simulink model "RotatingMasses_Template"  (R2019b)
settings: Solver=ode1  StartTime=0.0  StopTime=110  FixedStep=0.002  RelTol=1e-3  EnableMultiTasking=on
PostLoadFcn:
  | qc_set_target_type(getConfigSet(bdroot, 'QUARC Default Target Configuration'));
values from neighbouring files (symbols this model uses):
  data = dataset_struct    [create_data.m]    (also in data_loader.m = [])
  deg_to_rad = pi/180    (= 0.0174532925199)    [sensors_parameters.m]
  experiment = merge( experiment, experiment2 )    [blackbox_est.m]    (also in experiment_handler.m = obj.experiments{idx_exp}; guided_script.m = e_h.experiments{40}; test_controllori.m = e_h.load_experiment)
  pulse_to_rad = 2*pi/pulse_per_rev_encoder    (= 0.00153398078789)    [sensors_parameters.m]
  V_th = V_max*1    [sensors_parameters.m]
  Vmin_pot = -4.8924    [sensors_parameters.m]
  volt_to_deg_potentiometer = 352/(Vmax_pot-Vmin_pot)    (= 36.7512711555)    [sensors_parameters.m]
undefined symbols (not defined in the file or in its folder): controller, HIL, qc_get_step_size
libraries: simulink x43, cstblocks x15, quarc_library x5
(part 2 of 3)

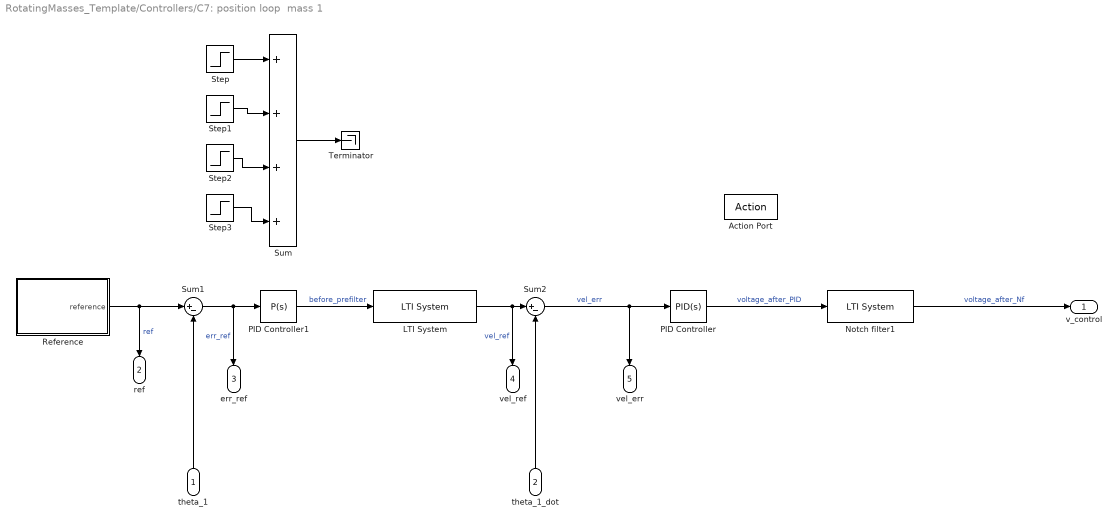
== system RotatingMasses_Template/Controllers/C7: position loop  mass 1 ==
  theta_1 : Inport
  theta_1_dot : Inport  Port=2
  Action Port : ActionPort  ActionPortLabel=elseif( u1==7)
  LTI System : cstblocks/LTI System  sys=controller.c7.Pf  IC=[]
  Notch filter1 : cstblocks/LTI System  sys=controller.c7.Nf  IC=[]
  PID Controller : simulink/Continuous/PID Controller  Controller=PID  Form=Parallel  TimeDomain=Continuous-time  SampleTime=-1  IntegratorMethod=Forward Euler  FilterMethod=Forward Euler  ControllerParametersSource=internal  P=controller.c7.Kp  I=controller.c7.Ki  D=controller.c7.Kd  UseFilter=on  N=100  TunerSelectOption=Transfer Function Based (PID Tuner App)  InitialConditionSource=internal  InitialConditionForIntegrator=0  InitialConditionForFilter=0  DifferentiatorICPrevScaledInput=0  ExternalReset=none  TrackingMode=off  Kt=1  LimitOutput=on  UpperSaturationLimit=10  LowerSaturationLimit=-10  LinearizeAsGain=on  AntiWindupMode=clamping  Kb=1  POutMin=[]  POutMax=[]  IOutMin=[]  IOutMax=[]  DOutMin=[]  DOutMax=[]  NOutMin=[]  NOutMax=[]  SumOutMin=[]  SumOutMax=[]  SaturationOutMin=[]  SaturationOutMax=[]  PParamMin=[]  PParamMax=[]  IParamMin=[]  IParamMax=[]  DParamMin=[]  DParamMax=[]  NParamMin=[]  NParamMax=[]  KbParamMin=[]  KbParamMax=[]  KtParamMin=[]  KtParamMax=[]  KbOutMin=[]  KbOutMax=[]  KtOutMin=[]  KtOutMax=[]  IntegratorOutMin=[]  IntegratorOutMax=[]  FilterOutMin=[]  FilterOutMax=[]  SumI1OutMin=[]  SumI1OutMax=[]  SumI2OutMin=[]  SumI2OutMax=[]  SumI3OutMin=[]  SumI3OutMax=[]  SumI4OutMin=[]  SumI4OutMax=[]  SumDOutMin=[]  SumDOutMax=[]  DifferentiatorOutMin=[]  DifferentiatorOutMax=[]  FilterDiffOutCoefMin=[]  FilterDiffOutCoefMax=[]  ReciprocalOutMin=[]  ReciprocalOutMax=[]  SumDenOutMin=[]  SumDenOutMax=[]  SumNumOutMin=[]  SumNumOutMax=[]  DivideOutMin=[]  DivideOutMax=[]  IntegratorContinuousStateAttributes=''  IntegratorStateMustResolveToSignalObject=off  IntegratorRTWStateStorageClass=Auto  FilterContinuousStateAttributes=''  FilterStateMustResolveToSignalObject=off  FilterRTWStateStorageClass=Auto  ParallelPVariant=InternalParameters  IdealPVariant=Disabled  IVariant=InternalParameters  DVariant=InternalParameters  IntegratorVariant=Continuous  SatVariant=Enabled  AWVariant=ContClampingParallel  PCopyVariant=Disabled  TRVariant=Disabled  FdbkBlocksVariant=Forward  IdealPFdbkVariant=Disabled  SatFdbkVariant=Disabled  DerivativeFilterVariant=ContFilter  NVariant=InternalParameters  NCopyVariant=Disabled  FilterICVariant=InternalICsFilter  IntegratorICVariant=InternalICs  ExternalResetVariant=Disabled  TRSumVariant=Passthrough  SumFdbkVariant=Disabled  SumVariant=Sum_PID
  PID Controller1 : simulink/Continuous/PID Controller  Controller=P  Form=Parallel  TimeDomain=Continuous-time  SampleTime=-1  IntegratorMethod=Forward Euler  FilterMethod=Forward Euler  ControllerParametersSource=internal  P=controller.c7.kp_p  I=controller.c6.Ki  D=controller.c6.Kd  UseFilter=on  N=100  TunerSelectOption=Transfer Function Based (PID Tuner App)  InitialConditionSource=internal  InitialConditionForIntegrator=0  InitialConditionForFilter=0  DifferentiatorICPrevScaledInput=0  ExternalReset=none  TrackingMode=off  Kt=1  LimitOutput=on  UpperSaturationLimit=10  LowerSaturationLimit=-10  LinearizeAsGain=on  AntiWindupMode=clamping  Kb=1  POutMin=[]  POutMax=[]  IOutMin=[]  IOutMax=[]  DOutMin=[]  DOutMax=[]  NOutMin=[]  NOutMax=[]  SumOutMin=[]  SumOutMax=[]  SaturationOutMin=[]  SaturationOutMax=[]  PParamMin=[]  PParamMax=[]  IParamMin=[]  IParamMax=[]  DParamMin=[]  DParamMax=[]  NParamMin=[]  NParamMax=[]  KbParamMin=[]  KbParamMax=[]  KtParamMin=[]  KtParamMax=[]  KbOutMin=[]  KbOutMax=[]  KtOutMin=[]  KtOutMax=[]  IntegratorOutMin=[]  IntegratorOutMax=[]  FilterOutMin=[]  FilterOutMax=[]  SumI1OutMin=[]  SumI1OutMax=[]  SumI2OutMin=[]  SumI2OutMax=[]  SumI3OutMin=[]  SumI3OutMax=[]  SumI4OutMin=[]  SumI4OutMax=[]  SumDOutMin=[]  SumDOutMax=[]  DifferentiatorOutMin=[]  DifferentiatorOutMax=[]  FilterDiffOutCoefMin=[]  FilterDiffOutCoefMax=[]  ReciprocalOutMin=[]  ReciprocalOutMax=[]  SumDenOutMin=[]  SumDenOutMax=[]  SumNumOutMin=[]  SumNumOutMax=[]  DivideOutMin=[]  DivideOutMax=[]  IntegratorContinuousStateAttributes=''  IntegratorStateMustResolveToSignalObject=off  IntegratorRTWStateStorageClass=Auto  FilterContinuousStateAttributes=''  FilterStateMustResolveToSignalObject=off  FilterRTWStateStorageClass=Auto  ParallelPVariant=InternalParameters  IdealPVariant=Disabled  IVariant=Disabled  DVariant=Disabled  IntegratorVariant=Disabled  SatVariant=Enabled  AWVariant=Disabled  PCopyVariant=Disabled  TRVariant=Disabled  FdbkBlocksVariant=Forward  IdealPFdbkVariant=Disabled  SatFdbkVariant=Disabled  DerivativeFilterVariant=Disabled  NVariant=Disabled  NCopyVariant=Disabled_SignalSpec  FilterICVariant=Disabled  IntegratorICVariant=Disabled  ExternalResetVariant=Disabled  TRSumVariant=Passthrough  SumFdbkVariant=Disabled  SumVariant=Passthrough_P
  Reference : Subsystem
  Step : Step  After=pi/4  SampleTime=0
  Step1 : Step  Time=10  After=-2*pi-pi/4  SampleTime=0
  Step2 : Step  Time=20  After=2*pi  SampleTime=0
  Step3 : Step  Time=30  After=6*pi  SampleTime=0
  Sum : Sum  Inputs=++++
  Sum1 : Sum  Inputs=|+-
  Sum2 : Sum  Inputs=|+-
  Terminator : Terminator
  v_control : Outport
  "ref " : Outport  Port=2
  "err_ref " : Outport  Port=3
  vel_ref : Outport  Port=4
  vel_err : Outport  Port=5
  wires:
  Notch filter1/1 -> v_control/1  "voltage_after_Nf"
  LTI System/1 -> vel_ref/1, Sum2/1  "vel_ref"
  Reference/1(reference) -> Sum1/1, "ref "/1  "ref"
  theta_1_dot/1 -> Sum2/2
  PID Controller/1 -> Notch filter1/1  "voltage_after_PID"
  Sum2/1 -> PID Controller/1, vel_err/1  "vel_err"
  theta_1/1 -> Sum1/2
  Sum1/1 -> PID Controller1/1, "err_ref "/1  "err_ref"
  PID Controller1/1 -> LTI System/1  "before_prefilter"
  Step2/1 -> Sum/3
  Step3/1 -> Sum/4
  Step1/1 -> Sum/2
  Step/1 -> Sum/1
  Sum/1 -> Terminator/1

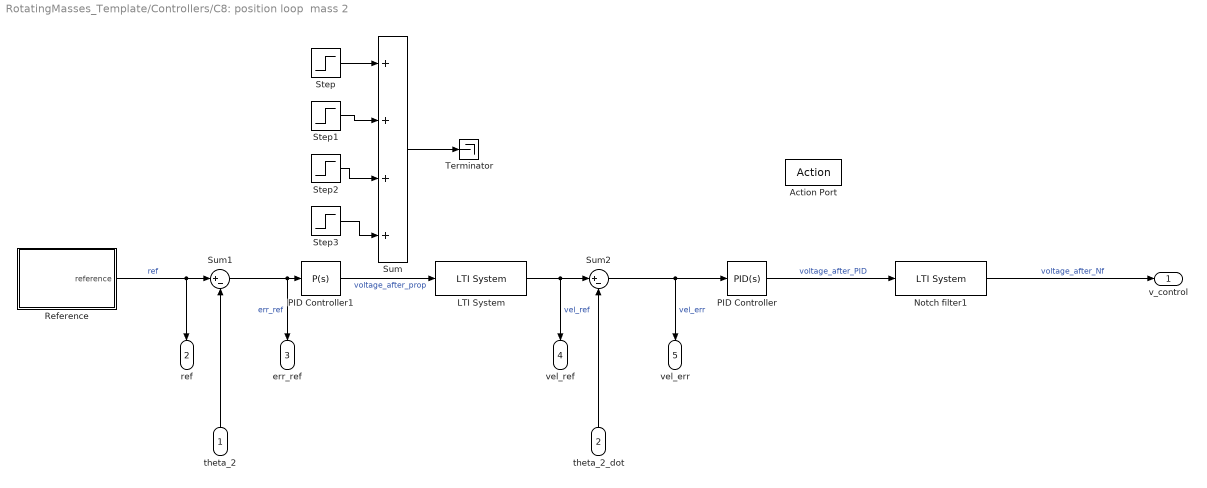
== system RotatingMasses_Template/Controllers/C8: position loop  mass 2 ==
  theta_2 : Inport
  theta_2_dot : Inport  Port=2
  Action Port : ActionPort  ActionPortLabel=elseif( u1==8)
  LTI System : cstblocks/LTI System  sys=controller.c8.Pf  IC=[]
  Notch filter1 : cstblocks/LTI System  sys=controller.c8.Nf  IC=[]
  PID Controller : simulink/Continuous/PID Controller  Controller=PID  Form=Parallel  TimeDomain=Continuous-time  SampleTime=-1  IntegratorMethod=Forward Euler  FilterMethod=Forward Euler  ControllerParametersSource=internal  P=controller.c8.Kp  I=controller.c8.Ki  D=controller.c8.Kd  UseFilter=on  N=100  TunerSelectOption=Transfer Function Based (PID Tuner App)  InitialConditionSource=internal  InitialConditionForIntegrator=0  InitialConditionForFilter=0  DifferentiatorICPrevScaledInput=0  ExternalReset=none  TrackingMode=off  Kt=1  LimitOutput=on  UpperSaturationLimit=10  LowerSaturationLimit=-10  LinearizeAsGain=on  AntiWindupMode=clamping  Kb=1  POutMin=[]  POutMax=[]  IOutMin=[]  IOutMax=[]  DOutMin=[]  DOutMax=[]  NOutMin=[]  NOutMax=[]  SumOutMin=[]  SumOutMax=[]  SaturationOutMin=[]  SaturationOutMax=[]  PParamMin=[]  PParamMax=[]  IParamMin=[]  IParamMax=[]  DParamMin=[]  DParamMax=[]  NParamMin=[]  NParamMax=[]  KbParamMin=[]  KbParamMax=[]  KtParamMin=[]  KtParamMax=[]  KbOutMin=[]  KbOutMax=[]  KtOutMin=[]  KtOutMax=[]  IntegratorOutMin=[]  IntegratorOutMax=[]  FilterOutMin=[]  FilterOutMax=[]  SumI1OutMin=[]  SumI1OutMax=[]  SumI2OutMin=[]  SumI2OutMax=[]  SumI3OutMin=[]  SumI3OutMax=[]  SumI4OutMin=[]  SumI4OutMax=[]  SumDOutMin=[]  SumDOutMax=[]  DifferentiatorOutMin=[]  DifferentiatorOutMax=[]  FilterDiffOutCoefMin=[]  FilterDiffOutCoefMax=[]  ReciprocalOutMin=[]  ReciprocalOutMax=[]  SumDenOutMin=[]  SumDenOutMax=[]  SumNumOutMin=[]  SumNumOutMax=[]  DivideOutMin=[]  DivideOutMax=[]  IntegratorContinuousStateAttributes=''  IntegratorStateMustResolveToSignalObject=off  IntegratorRTWStateStorageClass=Auto  FilterContinuousStateAttributes=''  FilterStateMustResolveToSignalObject=off  FilterRTWStateStorageClass=Auto  ParallelPVariant=InternalParameters  IdealPVariant=Disabled  IVariant=InternalParameters  DVariant=InternalParameters  IntegratorVariant=Continuous  SatVariant=Enabled  AWVariant=ContClampingParallel  PCopyVariant=Disabled  TRVariant=Disabled  FdbkBlocksVariant=Forward  IdealPFdbkVariant=Disabled  SatFdbkVariant=Disabled  DerivativeFilterVariant=ContFilter  NVariant=InternalParameters  NCopyVariant=Disabled  FilterICVariant=InternalICsFilter  IntegratorICVariant=InternalICs  ExternalResetVariant=Disabled  TRSumVariant=Passthrough  SumFdbkVariant=Disabled  SumVariant=Sum_PID
  PID Controller1 : simulink/Continuous/PID Controller  Controller=P  Form=Parallel  TimeDomain=Continuous-time  SampleTime=-1  IntegratorMethod=Forward Euler  FilterMethod=Forward Euler  ControllerParametersSource=internal  P=controller.c8.kp_p  I=controller.c6.Ki  D=controller.c6.Kd  UseFilter=on  N=100  TunerSelectOption=Transfer Function Based (PID Tuner App)  InitialConditionSource=internal  InitialConditionForIntegrator=0  InitialConditionForFilter=0  DifferentiatorICPrevScaledInput=0  ExternalReset=none  TrackingMode=off  Kt=1  LimitOutput=on  UpperSaturationLimit=10  LowerSaturationLimit=-10  LinearizeAsGain=on  AntiWindupMode=clamping  Kb=1  POutMin=[]  POutMax=[]  IOutMin=[]  IOutMax=[]  DOutMin=[]  DOutMax=[]  NOutMin=[]  NOutMax=[]  SumOutMin=[]  SumOutMax=[]  SaturationOutMin=[]  SaturationOutMax=[]  PParamMin=[]  PParamMax=[]  IParamMin=[]  IParamMax=[]  DParamMin=[]  DParamMax=[]  NParamMin=[]  NParamMax=[]  KbParamMin=[]  KbParamMax=[]  KtParamMin=[]  KtParamMax=[]  KbOutMin=[]  KbOutMax=[]  KtOutMin=[]  KtOutMax=[]  IntegratorOutMin=[]  IntegratorOutMax=[]  FilterOutMin=[]  FilterOutMax=[]  SumI1OutMin=[]  SumI1OutMax=[]  SumI2OutMin=[]  SumI2OutMax=[]  SumI3OutMin=[]  SumI3OutMax=[]  SumI4OutMin=[]  SumI4OutMax=[]  SumDOutMin=[]  SumDOutMax=[]  DifferentiatorOutMin=[]  DifferentiatorOutMax=[]  FilterDiffOutCoefMin=[]  FilterDiffOutCoefMax=[]  ReciprocalOutMin=[]  ReciprocalOutMax=[]  SumDenOutMin=[]  SumDenOutMax=[]  SumNumOutMin=[]  SumNumOutMax=[]  DivideOutMin=[]  DivideOutMax=[]  IntegratorContinuousStateAttributes=''  IntegratorStateMustResolveToSignalObject=off  IntegratorRTWStateStorageClass=Auto  FilterContinuousStateAttributes=''  FilterStateMustResolveToSignalObject=off  FilterRTWStateStorageClass=Auto  ParallelPVariant=InternalParameters  IdealPVariant=Disabled  IVariant=Disabled  DVariant=Disabled  IntegratorVariant=Disabled  SatVariant=Enabled  AWVariant=Disabled  PCopyVariant=Disabled  TRVariant=Disabled  FdbkBlocksVariant=Forward  IdealPFdbkVariant=Disabled  SatFdbkVariant=Disabled  DerivativeFilterVariant=Disabled  NVariant=Disabled  NCopyVariant=Disabled_SignalSpec  FilterICVariant=Disabled  IntegratorICVariant=Disabled  ExternalResetVariant=Disabled  TRSumVariant=Passthrough  SumFdbkVariant=Disabled  SumVariant=Passthrough_P
  Reference : Subsystem
  Step : Step  After=pi/4  SampleTime=0
  Step1 : Step  Time=10  After=-2*pi-pi/4  SampleTime=0
  Step2 : Step  Time=20  After=2*pi  SampleTime=0
  Step3 : Step  Time=30  After=6*pi  SampleTime=0
  Sum : Sum  Inputs=++++
  Sum1 : Sum  Inputs=|+-
  Sum2 : Sum  Inputs=|+-
  Terminator : Terminator
  v_control : Outport
  "ref " : Outport  Port=2
  "err_ref " : Outport  Port=3
  vel_ref : Outport  Port=4
  vel_err : Outport  Port=5
  wires:
  theta_2_dot/1 -> Sum2/2
  PID Controller/1 -> Notch filter1/1  "voltage_after_PID"
  Notch filter1/1 -> v_control/1  "voltage_after_Nf"
  LTI System/1 -> vel_ref/1, Sum2/1  "vel_ref"
  theta_2/1 -> Sum1/2
  Sum1/1 -> "err_ref "/1, PID Controller1/1  "err_ref"
  Sum2/1 -> PID Controller/1, vel_err/1  "vel_err"
  PID Controller1/1 -> LTI System/1  "voltage_after_prop"
  Step2/1 -> Sum/3
  Step3/1 -> Sum/4
  Step1/1 -> Sum/2
  Step/1 -> Sum/1
  Reference/1(reference) -> Sum1/1, "ref "/1  "ref"
  Sum/1 -> Terminator/1

== system RotatingMasses_Template/Controllers/C9: Pole placement + observer 1dof, speed ==
  theta_1_dot : Inport
  x_1_dof : Inport  Port=2
  Action Port : ActionPort  ActionPortLabel=elseif( u1 == 9)
  Constant : Constant  Value=2
  Integrator : Integrator
  K_v : Gain  Gain=controller.c9.K_v*0
  Pole placement : Gain  Gain=controller.c9.K_x  Multiplication=Matrix(K*u)
  Reference : Subsystem
  Sum : Sum  Inputs=--|
  Sum2 : Sum  Inputs=|+-
  voltage : Outport
  ref : Outport  Port=2
  err_ref : Outport  Port=3
  wires:
  Pole placement/1 -> Sum/2  "voltage_pp"
  Sum/1 -> voltage/1
  Integrator/1 -> K_v/1
  Sum2/1 -> err_ref/1, Integrator/1  "err_ref"
  Reference/1(reference) -> ref/1, Sum2/1
  theta_1_dot/1 -> Sum2/2
  x_1_dof/1 -> Pole placement/1
  Constant/1 -> Sum/1

== system RotatingMasses_Template/Controllers/Reference ==
  Action Port : ActionPort  ActionPortLabel=if(u1 == 0)
  Clock : Clock
  Constant : Constant  Value=experiment.step.init_time
  Constant1 : Constant  Value=experiment.step.step_size
  Gain : Gain  Gain=experiment.sinesweep.v_max-experiment.sinesweep.mean_value
  MATLAB Function : MATLAB Function  TreatAsAtomicUnit=on
  Sum1 : Sum  Inputs=+++
  Sum2 : Sum  Inputs=|++
  Switch : Switch  Criteria=u2 > Threshold
  interrupt_time : Step  Time=experiment.sinesweep.target_time  Before=1  After=-1  SampleTime=0
  lower_limit : Saturate  UpperLimit=max( experiment.ramp.init_value, experiment.ramp.final_value )  LowerLimit=min( experiment.ramp.init_value, experiment.ramp.final_value )
  mean_value : Constant  Value=experiment.sinesweep.mean_value
  ramp_decreasing : simulink/Sources/Ramp  slope=experiment.ramp.ramp_pend  start=experiment.ramp.init_time  InitialOutput=experiment.ramp.init_value
  security_stop : Constant  Value=0
  sine_sweep : simulink/Sources/Chirp Signal  f1=experiment.sinesweep.init_freq  T=experiment.sinesweep.target_time  f2=experiment.sinesweep.final_freq
  reference : Outport
  wires:
  mean_value/1 -> Sum2/1
  lower_limit/1 -> Sum1/2  "ramp"
  Switch/1 -> Sum2/2
  interrupt_time/1 -> Switch/2
  Sum2/1 -> Sum1/3  "sinesweep"
  Sum1/1 -> reference/1  "reference"
  security_stop/1 -> Switch/3
  ramp_decreasing/1 -> lower_limit/1
  Gain/1 -> Switch/1
  sine_sweep/1 -> Gain/1
  Clock/1 -> MATLAB Function/3(t)
  Constant/1 -> MATLAB Function/1(i_t)
  Constant1/1 -> MATLAB Function/2(s_a)
  MATLAB Function/1(step) -> Sum1/1  "step"

== system RotatingMasses_Template/Controllers/1dof Observers/Red_obs_1dof ==
  u : Inport
  y1: theta_l : Inport  Port=2
  y2: theta_1 : Inport  Port=3
  Gain : Gain  Gain=controller.red_obs_1dof.L  Multiplication=Matrix(K*u)
  Gain1 : Gain  Gain=-1
  Mux : Mux  Inputs=3
  Mux1 : Mux  Inputs=2
  Mux2 : Mux  Inputs=2
  Observer : StateSpace  A=controller.red_obs_1dof.A  B=controller.red_obs_1dof.B  C=controller.red_obs_1dof.C  D=controller.red_obs_1dof.D  InitialCondition=[data.motor_pos_0;0]
  Sum1 : Sum  Inputs=|++
  x : Outport
  wires:
  Mux2/1 -> x/1  "x"
  u/1 -> Mux/1
  Gain1/1 -> Mux2/2  "theta_1, theta_1_dot"
  y2: theta_1/1 -> Mux/3, Mux1/2
  Gain/1 -> Sum1/2
  Mux1/1 -> Gain/1, Gain1/1  "y"
  y1: theta_l/1 -> Mux/2, Mux1/1
  Mux/1 -> Observer/1
  Sum1/1 -> Mux2/1  "theta_l, theta_l_dot"
  Observer/1 -> Sum1/1

== system RotatingMasses_Template/Controllers/1dof Observers/obs_1_dof ==
  u : Inport
  y1: theta_l : Inport  Port=2
  y2: theta_1 : Inport  Port=3
  Mux : Mux  Inputs=3
  Observer : StateSpace  A=controller.obs_1dof.A  B=controller.obs_1dof.B  C=controller.obs_1dof.C  D=controller.obs_1dof.D  InitialCondition=[]
  x : Outport
  wires:
  Mux/1 -> Observer/1
  u/1 -> Mux/1
  y1: theta_l/1 -> Mux/2
  y2: theta_1/1 -> Mux/3
  Observer/1 -> x/1  "x"

== system RotatingMasses_Template/Controllers/2dof Observers/Observer_2dof ==
  u : Inport
  y1: theta_l : Inport  Port=2
  y2: theta_1 : Inport  Port=3
  y3: theta_2 : Inport  Port=4
  Mux : Mux
  Observer : StateSpace  A=controller.obs_2dof.A  B=controller.obs_2dof.B  C=controller.obs_2dof.C  D=controller.obs_2dof.D  InitialCondition=[]
  x_2_dof : Outport
  wires:
  Observer/1 -> x_2_dof/1
  y1: theta_l/1 -> Mux/2
  u/1 -> Mux/1
  y3: theta_2/1 -> Mux/4
  Mux/1 -> Observer/1
  y2: theta_1/1 -> Mux/3

== system RotatingMasses_Template/Controllers/2dof Observers/red_obs_2dof ==
  u : Inport
  y1: theta_1 : Inport  Port=2
  y2: theta_1_dot : Inport  Port=3
  y3: theta_2 : Inport  Port=4
  y4: theta_2_dot : Inport  Port=5
  Gain : Gain  Gain=controller.red_obs_2dof.L  Multiplication=Matrix(K*u)
  Gain1 : Gain  Gain=-1
  Mux : Mux  Inputs=5
  Mux1 : Mux
  Mux2 : Mux  Inputs=2
  Observer : StateSpace  A=controller.red_obs_2dof.A  B=controller.red_obs_2dof.B  C=controller.red_obs_2dof.C  D=controller.red_obs_2dof.D  InitialCondition=[data.motor_pos_0;0]
  Sum1 : Sum  Inputs=|++
  x_2dof : Outport
  wires:
  Sum1/1 -> Mux2/1  "theta_l, theta_l_dot"
  y1: theta_1/1 -> Mux1/1, Mux/2
  Mux/1 -> Observer/1
  Observer/1 -> Sum1/1
  y2: theta_1_dot/1 -> Mux1/2, Mux/3
  y3: theta_2/1 -> Mux1/3, Mux/4
  Mux1/1 -> Gain/1, Gain1/1  "y"
  u/1 -> Mux/1
  y4: theta_2_dot/1 -> Mux1/4, Mux/5
  Gain/1 -> Sum1/2
  Gain1/1 -> Mux2/2  "theta_1, theta_1_dot, theta_2, theta_2_dot"
  Mux2/1 -> x_2dof/1  "x"

== system RotatingMasses_Template/Controllers/C10: Pole placement + observer 1dof, pos/Reference ==
  Clock : Clock
  Constant : Constant  Value=experiment.step.init_time
  Constant1 : Constant  Value=experiment.step.step_size
  Gain : Gain  Gain=experiment.sinesweep.v_max-experiment.sinesweep.mean_value
  MATLAB Function : MATLAB Function  TreatAsAtomicUnit=on
  Sum1 : Sum  Inputs=+++
  Sum2 : Sum  Inputs=|++
  Switch : Switch  Criteria=u2 > Threshold
  interrupt_time : Step  Time=experiment.sinesweep.target_time  Before=1  After=-1  SampleTime=0
  lower_limit : Saturate  UpperLimit=max( experiment.ramp.init_value, experiment.ramp.final_value )  LowerLimit=min( experiment.ramp.init_value, experiment.ramp.final_value )
  mean_value : Constant  Value=experiment.sinesweep.mean_value
  ramp_decreasing : simulink/Sources/Ramp  slope=experiment.ramp.ramp_pend  start=experiment.ramp.init_time  InitialOutput=experiment.ramp.init_value
  security_stop : Constant  Value=0
  sine_sweep : simulink/Sources/Chirp Signal  f1=experiment.sinesweep.init_freq  T=experiment.sinesweep.target_time  f2=experiment.sinesweep.final_freq
  reference : Outport
  wires:
  mean_value/1 -> Sum2/1
  lower_limit/1 -> Sum1/2  "ramp"
  Switch/1 -> Sum2/2
  interrupt_time/1 -> Switch/2
  Sum2/1 -> Sum1/3  "sinesweep"
  Sum1/1 -> reference/1  "reference"
  security_stop/1 -> Switch/3
  ramp_decreasing/1 -> lower_limit/1
  Gain/1 -> Switch/1
  sine_sweep/1 -> Gain/1
  Clock/1 -> MATLAB Function/3(t)
  Constant/1 -> MATLAB Function/1(i_t)
  Constant1/1 -> MATLAB Function/2(s_a)
  MATLAB Function/1(step) -> Sum1/1  "step"

== system RotatingMasses_Template/Controllers/C11: Pole placement + observer 2dof, speed/Reference ==
  Clock : Clock
  Constant : Constant  Value=experiment.step.init_time
  Constant1 : Constant  Value=experiment.step.step_size
  Gain : Gain  Gain=experiment.sinesweep.v_max-experiment.sinesweep.mean_value
  MATLAB Function : MATLAB Function  TreatAsAtomicUnit=on
  Sum1 : Sum  Inputs=+++
  Sum2 : Sum  Inputs=|++
  Switch : Switch  Criteria=u2 > Threshold
  interrupt_time : Step  Time=experiment.sinesweep.target_time  Before=1  After=-1  SampleTime=0
  lower_limit : Saturate  UpperLimit=max( experiment.ramp.init_value, experiment.ramp.final_value )  LowerLimit=min( experiment.ramp.init_value, experiment.ramp.final_value )
  mean_value : Constant  Value=experiment.sinesweep.mean_value
  ramp_decreasing : simulink/Sources/Ramp  slope=experiment.ramp.ramp_pend  start=experiment.ramp.init_time  InitialOutput=experiment.ramp.init_value
  security_stop : Constant  Value=0
  sine_sweep : simulink/Sources/Chirp Signal  f1=experiment.sinesweep.init_freq  T=experiment.sinesweep.target_time  f2=experiment.sinesweep.final_freq
  reference : Outport
  wires:
  mean_value/1 -> Sum2/1
  lower_limit/1 -> Sum1/2  "ramp"
  Switch/1 -> Sum2/2
  interrupt_time/1 -> Switch/2
  Sum2/1 -> Sum1/3  "sinesweep"
  Sum1/1 -> reference/1  "reference"
  security_stop/1 -> Switch/3
  ramp_decreasing/1 -> lower_limit/1
  Gain/1 -> Switch/1
  sine_sweep/1 -> Gain/1
  Clock/1 -> MATLAB Function/3(t)
  Constant/1 -> MATLAB Function/1(i_t)
  Constant1/1 -> MATLAB Function/2(s_a)
  MATLAB Function/1(step) -> Sum1/1  "step"

== system RotatingMasses_Template/Controllers/C12: Pole placement + observer 2dof, pos/Reference ==
  Clock : Clock
  Constant : Constant  Value=experiment.step.init_time
  Constant1 : Constant  Value=experiment.step.step_size
  Gain : Gain  Gain=experiment.sinesweep.v_max-experiment.sinesweep.mean_value
  MATLAB Function : MATLAB Function  TreatAsAtomicUnit=on
  Sum1 : Sum  Inputs=+++
  Sum2 : Sum  Inputs=|++
  Switch : Switch  Criteria=u2 > Threshold
  interrupt_time : Step  Time=experiment.sinesweep.target_time  Before=1  After=-1  SampleTime=0
  lower_limit : Saturate  UpperLimit=max( experiment.ramp.init_value, experiment.ramp.final_value )  LowerLimit=min( experiment.ramp.init_value, experiment.ramp.final_value )
  mean_value : Constant  Value=experiment.sinesweep.mean_value
  ramp_decreasing : simulink/Sources/Ramp  slope=experiment.ramp.ramp_pend  start=experiment.ramp.init_time  InitialOutput=experiment.ramp.init_value
  security_stop : Constant  Value=0
  sine_sweep : simulink/Sources/Chirp Signal  f1=experiment.sinesweep.init_freq  T=experiment.sinesweep.target_time  f2=experiment.sinesweep.final_freq
  reference : Outport
  wires:
  mean_value/1 -> Sum2/1
  lower_limit/1 -> Sum1/2  "ramp"
  Switch/1 -> Sum2/2
  interrupt_time/1 -> Switch/2
  Sum2/1 -> Sum1/3  "sinesweep"
  Sum1/1 -> reference/1  "reference"
  security_stop/1 -> Switch/3
  ramp_decreasing/1 -> lower_limit/1
  Gain/1 -> Switch/1
  sine_sweep/1 -> Gain/1
  Clock/1 -> MATLAB Function/3(t)
  Constant/1 -> MATLAB Function/1(i_t)
  Constant1/1 -> MATLAB Function/2(s_a)
  MATLAB Function/1(step) -> Sum1/1  "step"

== system RotatingMasses_Template/Controllers/C13: Pole placement + red observer 1dof, speed1/Red_obs_1dof ==
  In1 : Inport
  In2 : Inport  Port=2
  In3 : Inport  Port=3
  Demux : Demux
  Gain : Gain  Gain=controller.red_obs_1dof.L  Multiplication=Matrix(K*u)
  Gain1 : Gain  Gain=-1
  Mux : Mux  Inputs=3
  Mux{1..4} (4 alike) : Mux  Inputs=2
  Observer : StateSpace  A=controller.red_obs_1dof.A  B=controller.red_obs_1dof.B  C=controller.red_obs_1dof.C  D=controller.red_obs_1dof.D  InitialCondition=[data.motor_pos_0;0]
  Scope : Scope  NumInputPorts=2
  Sum1 : Sum  Inputs=|++
  Terminator : Terminator
  Terminator1 : Terminator
  x : Outport
  wires:
  Mux2/1 -> x/1  "x"
  In2/1 -> Mux/1
  Mux3/1 -> Scope/1
  Mux4/1 -> Scope/2
  Demux/4 -> Mux4/1
  Gain1/1 -> Mux2/2  "theta_1, theta_1_dot"
  Demux/2 -> Terminator1/1
  In3/1 -> Mux/3, Mux4/2, Mux1/2
  Demux/1 -> Terminator/1
  Gain/1 -> Sum1/2
  Mux1/1 -> Gain/1, Gain1/1  "y"
  In1/1 -> Mux/2, Mux3/2, Mux1/1
  Mux/1 -> Observer/1
  Sum1/1 -> Mux2/1  "theta_l, theta_l_dot"
  Observer/1 -> Sum1/1, Demux/1
  Demux/3 -> Mux3/1

== system RotatingMasses_Template/Controllers/C13: Pole placement + red observer 1dof, speed1/Reference ==
  Clock : Clock
  Constant : Constant  Value=experiment.step.init_time
  Constant1 : Constant  Value=experiment.step.step_size
  Gain : Gain  Gain=experiment.sinesweep.v_max-experiment.sinesweep.mean_value
  MATLAB Function : MATLAB Function  TreatAsAtomicUnit=on
  Sum1 : Sum  Inputs=+++
  Sum2 : Sum  Inputs=|++
  Switch : Switch  Criteria=u2 > Threshold
  interrupt_time : Step  Time=experiment.sinesweep.target_time  Before=1  After=-1  SampleTime=0
  lower_limit : Saturate  UpperLimit=max( experiment.ramp.init_value, experiment.ramp.final_value )  LowerLimit=min( experiment.ramp.init_value, experiment.ramp.final_value )
  mean_value : Constant  Value=experiment.sinesweep.mean_value
  ramp_decreasing : simulink/Sources/Ramp  slope=experiment.ramp.ramp_pend  start=experiment.ramp.init_time  InitialOutput=experiment.ramp.init_value
  security_stop : Constant  Value=0
  sine_sweep : simulink/Sources/Chirp Signal  f1=experiment.sinesweep.init_freq  T=experiment.sinesweep.target_time  f2=experiment.sinesweep.final_freq
  reference : Outport
  wires:
  mean_value/1 -> Sum2/1
  lower_limit/1 -> Sum1/2  "ramp"
  Switch/1 -> Sum2/2
  interrupt_time/1 -> Switch/2
  Sum2/1 -> Sum1/3  "sinesweep"
  Sum1/1 -> reference/1  "reference"
  security_stop/1 -> Switch/3
  ramp_decreasing/1 -> lower_limit/1
  Gain/1 -> Switch/1
  sine_sweep/1 -> Gain/1
  Clock/1 -> MATLAB Function/3(t)
  Constant/1 -> MATLAB Function/1(i_t)
  Constant1/1 -> MATLAB Function/2(s_a)
  MATLAB Function/1(step) -> Sum1/1  "step"

== system RotatingMasses_Template/Controllers/C14: Pole placement + red observer 1dof, pos1/Reference ==
  Clock : Clock
  Constant : Constant  Value=experiment.step.init_time
  Constant1 : Constant  Value=experiment.step.step_size
  Gain : Gain  Gain=experiment.sinesweep.v_max-experiment.sinesweep.mean_value
  MATLAB Function : MATLAB Function  TreatAsAtomicUnit=on
  Sum1 : Sum  Inputs=+++
  Sum2 : Sum  Inputs=|++
  Switch : Switch  Criteria=u2 > Threshold
  interrupt_time : Step  Time=experiment.sinesweep.target_time  Before=1  After=-1  SampleTime=0
  lower_limit : Saturate  UpperLimit=max( experiment.ramp.init_value, experiment.ramp.final_value )  LowerLimit=min( experiment.ramp.init_value, experiment.ramp.final_value )
  mean_value : Constant  Value=experiment.sinesweep.mean_value
  ramp_decreasing : simulink/Sources/Ramp  slope=experiment.ramp.ramp_pend  start=experiment.ramp.init_time  InitialOutput=experiment.ramp.init_value
  security_stop : Constant  Value=0
  sine_sweep : simulink/Sources/Chirp Signal  f1=experiment.sinesweep.init_freq  T=experiment.sinesweep.target_time  f2=experiment.sinesweep.final_freq
  reference : Outport
  wires:
  mean_value/1 -> Sum2/1
  lower_limit/1 -> Sum1/2  "ramp"
  Switch/1 -> Sum2/2
  interrupt_time/1 -> Switch/2
  Sum2/1 -> Sum1/3  "sinesweep"
  Sum1/1 -> reference/1  "reference"
  security_stop/1 -> Switch/3
  ramp_decreasing/1 -> lower_limit/1
  Gain/1 -> Switch/1
  sine_sweep/1 -> Gain/1
  Clock/1 -> MATLAB Function/3(t)
  Constant/1 -> MATLAB Function/1(i_t)
  Constant1/1 -> MATLAB Function/2(s_a)
  MATLAB Function/1(step) -> Sum1/1  "step"

== system RotatingMasses_Template/Controllers/C15: Pole placement + observer 2dof, speed1/Reference ==
  Clock : Clock
  Constant : Constant  Value=experiment.step.init_time
  Constant1 : Constant  Value=experiment.step.step_size
  Gain : Gain  Gain=experiment.sinesweep.v_max-experiment.sinesweep.mean_value
  MATLAB Function : MATLAB Function  TreatAsAtomicUnit=on
  Sum1 : Sum  Inputs=+++
  Sum2 : Sum  Inputs=|++
  Switch : Switch  Criteria=u2 > Threshold
  interrupt_time : Step  Time=experiment.sinesweep.target_time  Before=1  After=-1  SampleTime=0
  lower_limit : Saturate  UpperLimit=max( experiment.ramp.init_value, experiment.ramp.final_value )  LowerLimit=min( experiment.ramp.init_value, experiment.ramp.final_value )
  mean_value : Constant  Value=experiment.sinesweep.mean_value
  ramp_decreasing : simulink/Sources/Ramp  slope=experiment.ramp.ramp_pend  start=experiment.ramp.init_time  InitialOutput=experiment.ramp.init_value
  security_stop : Constant  Value=0
  sine_sweep : simulink/Sources/Chirp Signal  f1=experiment.sinesweep.init_freq  T=experiment.sinesweep.target_time  f2=experiment.sinesweep.final_freq
  reference : Outport
  wires:
  mean_value/1 -> Sum2/1
  lower_limit/1 -> Sum1/2  "ramp"
  Switch/1 -> Sum2/2
  interrupt_time/1 -> Switch/2
  Sum2/1 -> Sum1/3  "sinesweep"
  Sum1/1 -> reference/1  "reference"
  security_stop/1 -> Switch/3
  ramp_decreasing/1 -> lower_limit/1
  Gain/1 -> Switch/1
  sine_sweep/1 -> Gain/1
  Clock/1 -> MATLAB Function/3(t)
  Constant/1 -> MATLAB Function/1(i_t)
  Constant1/1 -> MATLAB Function/2(s_a)
  MATLAB Function/1(step) -> Sum1/1  "step"

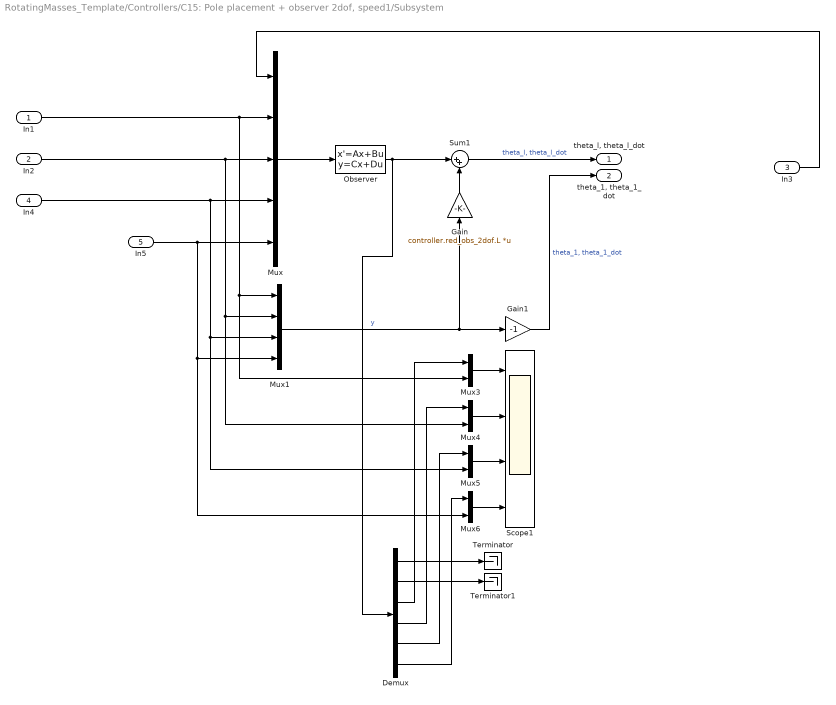
== system RotatingMasses_Template/Controllers/C15: Pole placement + observer 2dof, speed1/Subsystem ==
  In1 : Inport
  In2 : Inport  Port=2
  In3 : Inport  Port=3
  In4 : Inport  Port=4
  In5 : Inport  Port=5
  Demux : Demux  Outputs=6
  Gain : Gain  Gain=controller.red_obs_2dof.L  Multiplication=Matrix(K*u)
  Gain1 : Gain  Gain=-1
  Mux : Mux  Inputs=5
  Mux1 : Mux
  Mux{3..6} (4 alike) : Mux  Inputs=2
  Observer : StateSpace  A=controller.red_obs_2dof.A  B=controller.red_obs_2dof.B  C=controller.red_obs_2dof.C  D=controller.red_obs_2dof.D  InitialCondition=[data.motor_pos_0;0]
  Scope1 : Scope  NumInputPorts=4
  Sum1 : Sum  Inputs=|++
  Terminator : Terminator
  Terminator1 : Terminator
  "theta_l, theta_l_dot" : Outport
  "theta_1, theta_1_dot" : Outport  Port=2
  wires:
  Sum1/1 -> "theta_l, theta_l_dot"/1  "theta_l, theta_l_dot"
  Demux/3 -> Mux3/1
  Mux4/1 -> Scope1/2
  Demux/4 -> Mux4/1
  In1/1 -> Mux1/1, Mux3/2, Mux/2
  Demux/6 -> Mux6/1
  Mux5/1 -> Scope1/3
  Mux/1 -> Observer/1
  Observer/1 -> Demux/1, Sum1/1
  Demux/5 -> Mux5/1
  In2/1 -> Mux4/2, Mux1/2, Mux/3
  In4/1 -> Mux5/2, Mux1/3, Mux/4
  Mux6/1 -> Scope1/4
  Demux/2 -> Terminator1/1
  Mux1/1 -> Gain/1, Gain1/1  "y"
  In3/1 -> Mux/1
  In5/1 -> Mux6/2, Mux1/4, Mux/5
  Demux/1 -> Terminator/1
  Mux3/1 -> Scope1/1
  Gain/1 -> Sum1/2
  Gain1/1 -> "theta_1, theta_1_dot"/1  "theta_1, theta_1_dot"

== system RotatingMasses_Template/Controllers/C16: Pole placement + observer 2dof, pos1/Reference ==
  Clock : Clock
  Constant : Constant  Value=experiment.step.init_time
  Constant1 : Constant  Value=experiment.step.step_size
  Gain : Gain  Gain=experiment.sinesweep.v_max-experiment.sinesweep.mean_value
  MATLAB Function : MATLAB Function  TreatAsAtomicUnit=on
  Sum1 : Sum  Inputs=+++
  Sum2 : Sum  Inputs=|++
  Switch : Switch  Criteria=u2 > Threshold
  interrupt_time : Step  Time=experiment.sinesweep.target_time  Before=1  After=-1  SampleTime=0
  lower_limit : Saturate  UpperLimit=max( experiment.ramp.init_value, experiment.ramp.final_value )  LowerLimit=min( experiment.ramp.init_value, experiment.ramp.final_value )
  mean_value : Constant  Value=experiment.sinesweep.mean_value
  ramp_decreasing : simulink/Sources/Ramp  slope=experiment.ramp.ramp_pend  start=experiment.ramp.init_time  InitialOutput=experiment.ramp.init_value
  security_stop : Constant  Value=0
  sine_sweep : simulink/Sources/Chirp Signal  f1=experiment.sinesweep.init_freq  T=experiment.sinesweep.target_time  f2=experiment.sinesweep.final_freq
  reference : Outport
  wires:
  mean_value/1 -> Sum2/1
  lower_limit/1 -> Sum1/2  "ramp"
  Switch/1 -> Sum2/2
  interrupt_time/1 -> Switch/2
  Sum2/1 -> Sum1/3  "sinesweep"
  Sum1/1 -> reference/1  "reference"
  security_stop/1 -> Switch/3
  ramp_decreasing/1 -> lower_limit/1
  Gain/1 -> Switch/1
  sine_sweep/1 -> Gain/1
  Clock/1 -> MATLAB Function/3(t)
  Constant/1 -> MATLAB Function/1(i_t)
  Constant1/1 -> MATLAB Function/2(s_a)
  MATLAB Function/1(step) -> Sum1/1  "step"

== system RotatingMasses_Template/Controllers/C1: speed loop  mass 1/Reference ==
  Clock : Clock
  Constant : Constant  Value=experiment.step.init_time
  Constant1 : Constant  Value=experiment.step.step_size
  Gain : Gain  Gain=experiment.sinesweep.v_max-experiment.sinesweep.mean_value
  MATLAB Function : MATLAB Function  TreatAsAtomicUnit=on
  Sum1 : Sum  Inputs=+++
  Sum2 : Sum  Inputs=|++
  Switch : Switch  Criteria=u2 > Threshold
  interrupt_time : Step  Time=experiment.sinesweep.target_time  Before=1  After=-1  SampleTime=0
  lower_limit : Saturate  UpperLimit=max( experiment.ramp.init_value, experiment.ramp.final_value )  LowerLimit=min( experiment.ramp.init_value, experiment.ramp.final_value )
  mean_value : Constant  Value=experiment.sinesweep.mean_value
  ramp_decreasing : simulink/Sources/Ramp  slope=experiment.ramp.ramp_pend  start=experiment.ramp.init_time  InitialOutput=experiment.ramp.init_value
  security_stop : Constant  Value=0
  sine_sweep : simulink/Sources/Chirp Signal  f1=experiment.sinesweep.init_freq  T=experiment.sinesweep.target_time  f2=experiment.sinesweep.final_freq
  reference : Outport
  wires:
  mean_value/1 -> Sum2/1
  lower_limit/1 -> Sum1/2  "ramp"
  Switch/1 -> Sum2/2
  interrupt_time/1 -> Switch/2
  Sum2/1 -> Sum1/3  "sinesweep"
  Sum1/1 -> reference/1  "reference"
  security_stop/1 -> Switch/3
  ramp_decreasing/1 -> lower_limit/1
  Gain/1 -> Switch/1
  sine_sweep/1 -> Gain/1
  Clock/1 -> MATLAB Function/3(t)
  Constant/1 -> MATLAB Function/1(i_t)
  Constant1/1 -> MATLAB Function/2(s_a)
  MATLAB Function/1(step) -> Sum1/1  "step"

== system RotatingMasses_Template/Controllers/C1: speed loop  mass 1/Speed PI1 ==
  w_ref : Inport
  Add : Sum  Inputs=|++
  Gain : Gain  Gain=controller.c1.kp_v
  Saturation : Saturate  UpperLimit=V_th  LowerLimit=-V_th
  Transfer Fcn : TransferFcn  Denominator=[controller.c1.Ti_v 1]
  V_ref : Outport
  wires:
  Gain/1 -> Add/1
  Transfer Fcn/1 -> Add/2
  Saturation/1 -> V_ref/1, Transfer Fcn/1
  w_ref/1 -> Gain/1
  Add/1 -> Saturation/1

== system RotatingMasses_Template/Controllers/C2: position loop mass 1/Position P ==
  w_ref : Inport
  Gain : Gain  Gain=controller.c2.kp_p
  vel_ref : Outport
  wires:
  w_ref/1 -> Gain/1
  Gain/1 -> vel_ref/1

== system RotatingMasses_Template/Controllers/C2: position loop mass 1/Reference ==
  Clock : Clock
  Constant : Constant  Value=experiment.step.init_time
  Constant1 : Constant  Value=experiment.step.step_size
  Gain : Gain  Gain=experiment.sinesweep.v_max-experiment.sinesweep.mean_value
  MATLAB Function : MATLAB Function  TreatAsAtomicUnit=on
  Sum1 : Sum  Inputs=+++
  Sum2 : Sum  Inputs=|++
  Switch : Switch  Criteria=u2 > Threshold
  interrupt_time : Step  Time=experiment.sinesweep.target_time  Before=1  After=-1  SampleTime=0
  lower_limit : Saturate  UpperLimit=max( experiment.ramp.init_value, experiment.ramp.final_value )  LowerLimit=min( experiment.ramp.init_value, experiment.ramp.final_value )
  mean_value : Constant  Value=experiment.sinesweep.mean_value
  ramp_decreasing : simulink/Sources/Ramp  slope=experiment.ramp.ramp_pend  start=experiment.ramp.init_time  InitialOutput=experiment.ramp.init_value
  security_stop : Constant  Value=0
  sine_sweep : simulink/Sources/Chirp Signal  f1=experiment.sinesweep.init_freq  T=experiment.sinesweep.target_time  f2=experiment.sinesweep.final_freq
  reference : Outport
  wires:
  mean_value/1 -> Sum2/1
  lower_limit/1 -> Sum1/2  "ramp"
  Switch/1 -> Sum2/2
  interrupt_time/1 -> Switch/2
  Sum2/1 -> Sum1/3  "sinesweep"
  Sum1/1 -> reference/1  "reference"
  security_stop/1 -> Switch/3
  ramp_decreasing/1 -> lower_limit/1
  Gain/1 -> Switch/1
  sine_sweep/1 -> Gain/1
  Clock/1 -> MATLAB Function/3(t)
  Constant/1 -> MATLAB Function/1(i_t)
  Constant1/1 -> MATLAB Function/2(s_a)
  MATLAB Function/1(step) -> Sum1/1  "step"

== system RotatingMasses_Template/Controllers/C2: position loop mass 1/Speed PI + switch ==
  w_ref : Inport
  "Ti switch " : Inport  Port=2
  Abs : Abs
  Add : Sum  Inputs=|++
  Constant : Constant  Value=0
  Gain : Gain  Gain=controller.c2.kp_v
  Saturation : Saturate  UpperLimit=V_th  LowerLimit=-V_th
  Scope : Scope  NumInputPorts=2
  Switch : Switch  Criteria=u2 > Threshold  Threshold=10*pulse_to_rad
  Transfer Fcn : TransferFcn  Denominator=[controller.c2.Ti_v 1]
  V_ref : Outport
  wires:
  Gain/1 -> Add/1
  Transfer Fcn/1 -> Switch/1
  Saturation/1 -> Scope/2, V_ref/1, Transfer Fcn/1
  w_ref/1 -> Gain/1
  Add/1 -> Scope/1, Saturation/1
  Switch/1 -> Add/2
  Constant/1 -> Switch/3
  "Ti switch "/1 -> Abs/1
  Abs/1 -> Switch/2

== system RotatingMasses_Template/Controllers/C3: speed loop  mass 2/Reference ==
  Clock : Clock
  Constant : Constant  Value=experiment.step.init_time
  Constant1 : Constant  Value=experiment.step.step_size
  Gain : Gain  Gain=experiment.sinesweep.v_max-experiment.sinesweep.mean_value
  MATLAB Function : MATLAB Function  TreatAsAtomicUnit=on
  Sum1 : Sum  Inputs=+++
  Sum2 : Sum  Inputs=|++
  Switch : Switch  Criteria=u2 > Threshold
  interrupt_time : Step  Time=experiment.sinesweep.target_time  Before=1  After=-1  SampleTime=0
  lower_limit : Saturate  UpperLimit=max( experiment.ramp.init_value, experiment.ramp.final_value )  LowerLimit=min( experiment.ramp.init_value, experiment.ramp.final_value )
  mean_value : Constant  Value=experiment.sinesweep.mean_value
  ramp_decreasing : simulink/Sources/Ramp  slope=experiment.ramp.ramp_pend  start=experiment.ramp.init_time  InitialOutput=experiment.ramp.init_value
  security_stop : Constant  Value=0
  sine_sweep : simulink/Sources/Chirp Signal  f1=experiment.sinesweep.init_freq  T=experiment.sinesweep.target_time  f2=experiment.sinesweep.final_freq
  reference : Outport
  wires:
  mean_value/1 -> Sum2/1
  lower_limit/1 -> Sum1/2  "ramp"
  Switch/1 -> Sum2/2
  interrupt_time/1 -> Switch/2
  Sum2/1 -> Sum1/3  "sinesweep"
  Sum1/1 -> reference/1  "reference"
  security_stop/1 -> Switch/3
  ramp_decreasing/1 -> lower_limit/1
  Gain/1 -> Switch/1
  sine_sweep/1 -> Gain/1
  Clock/1 -> MATLAB Function/3(t)
  Constant/1 -> MATLAB Function/1(i_t)
  Constant1/1 -> MATLAB Function/2(s_a)
  MATLAB Function/1(step) -> Sum1/1  "step"

== system RotatingMasses_Template/Controllers/C3: speed loop  mass 2/Speed PI1 ==
  w_ref : Inport
  Add : Sum  Inputs=|++
  Gain : Gain  Gain=controller.c3.kp_v
  Saturation : Saturate  UpperLimit=V_th  LowerLimit=-V_th
  Transfer Fcn : TransferFcn  Denominator=[controller.c3.Ti_v 1]
  V_ref : Outport
  wires:
  Gain/1 -> Add/1
  Transfer Fcn/1 -> Add/2
  Saturation/1 -> V_ref/1, Transfer Fcn/1
  w_ref/1 -> Gain/1
  Add/1 -> Saturation/1

== system RotatingMasses_Template/Controllers/C4: position loop mass 2/Position P ==
  w_ref : Inport
  Gain : Gain  Gain=controller.c4.kp_p
  vel_ref : Outport
  wires:
  w_ref/1 -> Gain/1
  Gain/1 -> vel_ref/1

== system RotatingMasses_Template/Controllers/C4: position loop mass 2/Reference ==
  Clock : Clock
  Constant : Constant  Value=experiment.step.init_time
  Constant1 : Constant  Value=experiment.step.step_size
  Gain : Gain  Gain=experiment.sinesweep.v_max-experiment.sinesweep.mean_value
  MATLAB Function : MATLAB Function  TreatAsAtomicUnit=on
  Sum1 : Sum  Inputs=+++
  Sum2 : Sum  Inputs=|++
  Switch : Switch  Criteria=u2 > Threshold
  interrupt_time : Step  Time=experiment.sinesweep.target_time  Before=1  After=-1  SampleTime=0
  lower_limit : Saturate  UpperLimit=max( experiment.ramp.init_value, experiment.ramp.final_value )  LowerLimit=min( experiment.ramp.init_value, experiment.ramp.final_value )
  mean_value : Constant  Value=experiment.sinesweep.mean_value
  ramp_decreasing : simulink/Sources/Ramp  slope=experiment.ramp.ramp_pend  start=experiment.ramp.init_time  InitialOutput=experiment.ramp.init_value
  security_stop : Constant  Value=0
  sine_sweep : simulink/Sources/Chirp Signal  f1=experiment.sinesweep.init_freq  T=experiment.sinesweep.target_time  f2=experiment.sinesweep.final_freq
  reference : Outport
  wires:
  mean_value/1 -> Sum2/1
  lower_limit/1 -> Sum1/2  "ramp"
  Switch/1 -> Sum2/2
  interrupt_time/1 -> Switch/2
  Sum2/1 -> Sum1/3  "sinesweep"
  Sum1/1 -> reference/1  "reference"
  security_stop/1 -> Switch/3
  ramp_decreasing/1 -> lower_limit/1
  Gain/1 -> Switch/1
  sine_sweep/1 -> Gain/1
  Clock/1 -> MATLAB Function/3(t)
  Constant/1 -> MATLAB Function/1(i_t)
  Constant1/1 -> MATLAB Function/2(s_a)
  MATLAB Function/1(step) -> Sum1/1  "step"

== system RotatingMasses_Template/Controllers/C4: position loop mass 2/Speed PI + switch ==
  w_ref : Inport
  Ti control : Inport  Port=2
  Add : Sum  Inputs=|++
  Constant : Constant  Value=0
  Gain : Gain  Gain=controller.c4.kp_v
  Saturation : Saturate  UpperLimit=V_th  LowerLimit=-V_th
  Switch : Switch  Criteria=u2 > Threshold  Threshold=10*pulse_to_rad
  Transfer Fcn : TransferFcn  Denominator=[controller.c4.Ti_v 1]
  V_ref : Outport
  wires:
  Gain/1 -> Add/1
  Saturation/1 -> V_ref/1, Transfer Fcn/1
  Add/1 -> Saturation/1
  Transfer Fcn/1 -> Switch/1
  w_ref/1 -> Gain/1
  Constant/1 -> Switch/3
  Switch/1 -> Add/2
  Ti control/1 -> Switch/2

== system RotatingMasses_Template/Controllers/C5: speed loop  mass 1/Reference ==
  Clock : Clock
  Constant : Constant  Value=experiment.step.init_time
  Constant1 : Constant  Value=experiment.step.step_size
  Gain : Gain  Gain=experiment.sinesweep.v_max-experiment.sinesweep.mean_value
  MATLAB Function : MATLAB Function  TreatAsAtomicUnit=on
  Sum1 : Sum  Inputs=+++
  Sum2 : Sum  Inputs=|++
  Switch : Switch  Criteria=u2 > Threshold
  interrupt_time : Step  Time=experiment.sinesweep.target_time  Before=1  After=-1  SampleTime=0
  lower_limit : Saturate  UpperLimit=max( experiment.ramp.init_value, experiment.ramp.final_value )  LowerLimit=min( experiment.ramp.init_value, experiment.ramp.final_value )
  mean_value : Constant  Value=experiment.sinesweep.mean_value
  ramp_decreasing : simulink/Sources/Ramp  slope=experiment.ramp.ramp_pend  start=experiment.ramp.init_time  InitialOutput=experiment.ramp.init_value
  security_stop : Constant  Value=0
  sine_sweep : simulink/Sources/Chirp Signal  f1=experiment.sinesweep.init_freq  T=experiment.sinesweep.target_time  f2=experiment.sinesweep.final_freq
  reference : Outport
  wires:
  mean_value/1 -> Sum2/1
  lower_limit/1 -> Sum1/2  "ramp"
  Switch/1 -> Sum2/2
  interrupt_time/1 -> Switch/2
  Sum2/1 -> Sum1/3  "sinesweep"
  Sum1/1 -> reference/1  "reference"
  security_stop/1 -> Switch/3
  ramp_decreasing/1 -> lower_limit/1
  Gain/1 -> Switch/1
  sine_sweep/1 -> Gain/1
  Clock/1 -> MATLAB Function/3(t)
  Constant/1 -> MATLAB Function/1(i_t)
  Constant1/1 -> MATLAB Function/2(s_a)
  MATLAB Function/1(step) -> Sum1/1  "step"

== system RotatingMasses_Template/Controllers/C6: speed loop  mass 2/Reference ==
  Clock : Clock
  Constant : Constant  Value=experiment.step.init_time
  Constant1 : Constant  Value=experiment.step.step_size
  Gain : Gain  Gain=experiment.sinesweep.v_max-experiment.sinesweep.mean_value
  MATLAB Function : MATLAB Function  TreatAsAtomicUnit=on
  Sum1 : Sum  Inputs=+++
  Sum2 : Sum  Inputs=|++
  Switch : Switch  Criteria=u2 > Threshold
  interrupt_time : Step  Time=experiment.sinesweep.target_time  Before=1  After=-1  SampleTime=0
  lower_limit : Saturate  UpperLimit=max( experiment.ramp.init_value, experiment.ramp.final_value )  LowerLimit=min( experiment.ramp.init_value, experiment.ramp.final_value )
  mean_value : Constant  Value=experiment.sinesweep.mean_value
  ramp_decreasing : simulink/Sources/Ramp  slope=experiment.ramp.ramp_pend  start=experiment.ramp.init_time  InitialOutput=experiment.ramp.init_value
  security_stop : Constant  Value=0
  sine_sweep : simulink/Sources/Chirp Signal  f1=experiment.sinesweep.init_freq  T=experiment.sinesweep.target_time  f2=experiment.sinesweep.final_freq
  reference : Outport
  wires:
  mean_value/1 -> Sum2/1
  lower_limit/1 -> Sum1/2  "ramp"
  Switch/1 -> Sum2/2
  interrupt_time/1 -> Switch/2
  Sum2/1 -> Sum1/3  "sinesweep"
  Sum1/1 -> reference/1  "reference"
  security_stop/1 -> Switch/3
  ramp_decreasing/1 -> lower_limit/1
  Gain/1 -> Switch/1
  sine_sweep/1 -> Gain/1
  Clock/1 -> MATLAB Function/3(t)
  Constant/1 -> MATLAB Function/1(i_t)
  Constant1/1 -> MATLAB Function/2(s_a)
  MATLAB Function/1(step) -> Sum1/1  "step"

== system RotatingMasses_Template/Controllers/C7: position loop  mass 1/Reference ==
  Clock : Clock
  Constant : Constant  Value=experiment.step.init_time
  Constant1 : Constant  Value=experiment.step.step_size
  Gain : Gain  Gain=experiment.sinesweep.v_max-experiment.sinesweep.mean_value
  MATLAB Function : MATLAB Function  TreatAsAtomicUnit=on
  Sum1 : Sum  Inputs=+++
  Sum2 : Sum  Inputs=|++
  Switch : Switch  Criteria=u2 > Threshold
  interrupt_time : Step  Time=experiment.sinesweep.target_time  Before=1  After=-1  SampleTime=0
  lower_limit : Saturate  UpperLimit=max( experiment.ramp.init_value, experiment.ramp.final_value )  LowerLimit=min( experiment.ramp.init_value, experiment.ramp.final_value )
  mean_value : Constant  Value=experiment.sinesweep.mean_value
  ramp_decreasing : simulink/Sources/Ramp  slope=experiment.ramp.ramp_pend  start=experiment.ramp.init_time  InitialOutput=experiment.ramp.init_value
  security_stop : Constant  Value=0
  sine_sweep : simulink/Sources/Chirp Signal  f1=experiment.sinesweep.init_freq  T=experiment.sinesweep.target_time  f2=experiment.sinesweep.final_freq
  reference : Outport
  wires:
  mean_value/1 -> Sum2/1
  lower_limit/1 -> Sum1/2  "ramp"
  Switch/1 -> Sum2/2
  interrupt_time/1 -> Switch/2
  Sum2/1 -> Sum1/3  "sinesweep"
  Sum1/1 -> reference/1  "reference"
  security_stop/1 -> Switch/3
  ramp_decreasing/1 -> lower_limit/1
  Gain/1 -> Switch/1
  sine_sweep/1 -> Gain/1
  Clock/1 -> MATLAB Function/3(t)
  Constant/1 -> MATLAB Function/1(i_t)
  Constant1/1 -> MATLAB Function/2(s_a)
  MATLAB Function/1(step) -> Sum1/1  "step"

== system RotatingMasses_Template/Controllers/C8: position loop  mass 2/Reference ==
  Clock : Clock
  Constant : Constant  Value=experiment.step.init_time
  Constant1 : Constant  Value=experiment.step.step_size
  Gain : Gain  Gain=experiment.sinesweep.v_max-experiment.sinesweep.mean_value
  MATLAB Function : MATLAB Function  TreatAsAtomicUnit=on
  Sum1 : Sum  Inputs=+++
  Sum2 : Sum  Inputs=|++
  Switch : Switch  Criteria=u2 > Threshold
  interrupt_time : Step  Time=experiment.sinesweep.target_time  Before=1  After=-1  SampleTime=0
  lower_limit : Saturate  UpperLimit=max( experiment.ramp.init_value, experiment.ramp.final_value )  LowerLimit=min( experiment.ramp.init_value, experiment.ramp.final_value )
  mean_value : Constant  Value=experiment.sinesweep.mean_value
  ramp_decreasing : simulink/Sources/Ramp  slope=experiment.ramp.ramp_pend  start=experiment.ramp.init_time  InitialOutput=experiment.ramp.init_value
  security_stop : Constant  Value=0
  sine_sweep : simulink/Sources/Chirp Signal  f1=experiment.sinesweep.init_freq  T=experiment.sinesweep.target_time  f2=experiment.sinesweep.final_freq
  reference : Outport
  wires:
  mean_value/1 -> Sum2/1
  lower_limit/1 -> Sum1/2  "ramp"
  Switch/1 -> Sum2/2
  interrupt_time/1 -> Switch/2
  Sum2/1 -> Sum1/3  "sinesweep"
  Sum1/1 -> reference/1  "reference"
  security_stop/1 -> Switch/3
  ramp_decreasing/1 -> lower_limit/1
  Gain/1 -> Switch/1
  sine_sweep/1 -> Gain/1
  Clock/1 -> MATLAB Function/3(t)
  Constant/1 -> MATLAB Function/1(i_t)
  Constant1/1 -> MATLAB Function/2(s_a)
  MATLAB Function/1(step) -> Sum1/1  "step"

== system RotatingMasses_Template/Controllers/C9: Pole placement + observer 1dof, speed/Reference ==
  Clock : Clock
  Constant : Constant  Value=experiment.step.init_time
  Constant1 : Constant  Value=experiment.step.step_size
  Gain : Gain  Gain=experiment.sinesweep.v_max-experiment.sinesweep.mean_value
  MATLAB Function : MATLAB Function  TreatAsAtomicUnit=on
  Sum1 : Sum  Inputs=+++
  Sum2 : Sum  Inputs=|++
  Switch : Switch  Criteria=u2 > Threshold
  interrupt_time : Step  Time=experiment.sinesweep.target_time  Before=1  After=-1  SampleTime=0
  lower_limit : Saturate  UpperLimit=max( experiment.ramp.init_value, experiment.ramp.final_value )  LowerLimit=min( experiment.ramp.init_value, experiment.ramp.final_value )
  mean_value : Constant  Value=experiment.sinesweep.mean_value
  ramp_decreasing : simulink/Sources/Ramp  slope=experiment.ramp.ramp_pend  start=experiment.ramp.init_time  InitialOutput=experiment.ramp.init_value
  security_stop : Constant  Value=0
  sine_sweep : simulink/Sources/Chirp Signal  f1=experiment.sinesweep.init_freq  T=experiment.sinesweep.target_time  f2=experiment.sinesweep.final_freq
  reference : Outport
  wires:
  mean_value/1 -> Sum2/1
  lower_limit/1 -> Sum1/2  "ramp"
  Switch/1 -> Sum2/2
  interrupt_time/1 -> Switch/2
  Sum2/1 -> Sum1/3  "sinesweep"
  Sum1/1 -> reference/1  "reference"
  security_stop/1 -> Switch/3
  ramp_decreasing/1 -> lower_limit/1
  Gain/1 -> Switch/1
  sine_sweep/1 -> Gain/1
  Clock/1 -> MATLAB Function/3(t)
  Constant/1 -> MATLAB Function/1(i_t)
  Constant1/1 -> MATLAB Function/2(s_a)
  MATLAB Function/1(step) -> Sum1/1  "step"

== matlab function RotatingMasses_Template/encoder_raw_1/Reset and buffer count  ==
  settings: updateMethod=DISCRETE
  data: u input; y output
function y = fcn(u)
persistent oldu;
persistent buffer;
persistent oldy;
if isempty(oldu)
    oldu=0;
    oldy = 0;
    buffer = 0;
end
if u~=0 & oldu==0 %#ok<AND2>
    oldu=u;
end
y=u-oldu;
  
if ( y - oldy > 33000 )
    buffer = buffer-1;
elseif ( y - oldy < - 33000 )
    buffer = buffer+1;
end
oldy = y;

y = y + buffer*2^16;

== matlab function RotatingMasses_Template/encoder_raw_2/Reset and buffer count  ==
  settings: updateMethod=DISCRETE
  data: u input; y output
function y = fcn(u)
persistent oldu;
persistent buffer;
persistent oldy;
if isempty(oldu)
    oldu=0;
    oldy = 0;
    buffer = 0;
end
if u~=0 & oldu==0 %#ok<AND2>
    oldu=u;
end
y=u-oldu;
  
if ( y - oldy > 33000 )
    buffer = buffer-1;
elseif ( y - oldy < - 33000 )
    buffer = buffer+1;
end
oldy = y;

y = y + buffer*2^16;
